simulink model "GS_model"  (R2018b)
settings: Solver=ode5  StartTime=0.0  StopTime=SimuStopTime  FixedStep=T_Simu  RelTol=1e-3
InitFcn:
  | Initial
undefined symbols (not defined in the file or in its folder): Aba10, Aba20, aeroCIP2006_S, aeroCIP2006_X, aeroCIP2006_Y, Agl0, Ass_kS, Ass_n1, Ass_n2, Ass_n3, Ass_n4, Ass_Noise, Ass_R, Ass_Resolution, Ass_TmOrder, AssA_Fix_Abs, AssB_Fix_Abs, AssC_Fix_Abs, AssD_Fix_Abs, AssE_Fix_Aps, AssF_Fix_Aps, C, c_max, c_min, Cd, CenterOfFigNX, CenterOfFigNY, CenterOfFigNZ, CenterOfFigP1, CenterOfFigP2, CenterOfFigPX, CenterOfFigPY, CenterOfFigPZ, Cmu, Crou, DEG2RAD, DiscIntNeverNeededParam, Eg_Dir, Eg_F, Eg_PrepareTime, Eg_r_L_L, Fw_Abf, Fw_Hmax, Fw_J, Fw_Spd0, Fw_Tmax, git_hash_BaseLine, git_hash_Project, Gnss_Noise_Pos, Gnss_Noise_Vel, Gnss_PropgationTime, GyroA_Fix_Abg, GyroA_Noise, GyroB_Fix_Abg, GyroB_Noise, GyroC_Fix_Abg, GyroC_Noise, GyroD_Fix_Abg, GyroD_Noise, h ... (+94)
libraries: simulink x308, sharedutil x46, aerolibutil x37, sharedtransform x31, vrlib x14, aerolibgravity2 x2
(part 17 of 20)

== system GS_model/Subsystem2/Subsystem/Sensor/Gyro/GyroBModel/GyroErrSet/GyroErrSet/GyroErrSet_Jump/Triggered Subsystem8 ==
  In1 : Inport
  Enable : EnablePort
  Out1 : Outport
  wires:
  In1/1 -> Out1/1

== system GS_model/Subsystem2/Subsystem/Sensor/Gyro/GyroBModel/GyroErrSet/GyroErrSet/GyroErrSet_Wave/Triggered Subsystem1 ==
  In1 : Inport
  Enable : EnablePort
  Out1 : Outport
  wires:
  In1/1 -> Out1/1

== system GS_model/Subsystem2/Subsystem/Sensor/Gyro/GyroBModel/GyroErrSet/GyroErrSet/GyroErrSet_Wave/Triggered Subsystem2 ==
  In1 : Inport
  Enable : EnablePort
  Out1 : Outport
  wires:
  In1/1 -> Out1/1

== system GS_model/Subsystem2/Subsystem/Sensor/Gyro/GyroBModel/GyroErrSet/GyroErrSet/GyroErrSet_Wave/Triggered Subsystem8 ==
  In1 : Inport
  Enable : EnablePort
  Out1 : Outport
  wires:
  In1/1 -> Out1/1

== system GS_model/Subsystem2/Subsystem/Sensor/Gyro/GyroBModel/GyroErrSet/GyroErrSet/GyroErrSet_WildValue/Triggered Subsystem1 ==
  In1 : Inport
  Enable : EnablePort
  Out1 : Outport
  wires:
  In1/1 -> Out1/1

== system GS_model/Subsystem2/Subsystem/Sensor/Gyro/GyroBModel/GyroErrSet/GyroErrSet/GyroErrSet_WildValue/Triggered Subsystem2 ==
  In1 : Inport
  Enable : EnablePort
  Out1 : Outport
  wires:
  In1/1 -> Out1/1

== system GS_model/Subsystem2/Subsystem/Sensor/Gyro/GyroBModel/GyroErrSet/GyroErrSet/GyroErrSet_WildValue/Triggered Subsystem8 ==
  In1 : Inport
  Enable : EnablePort
  Out1 : Outport
  wires:
  In1/1 -> Out1/1

== system GS_model/Subsystem2/Subsystem/Sensor/Gyro/GyroCModel/GyroErrSet/GyroErrSet/GyroErrSet_Constant/Triggered Subsystem1 ==
  In1 : Inport
  Enable : EnablePort
  Out1 : Outport
  wires:
  In1/1 -> Out1/1

== system GS_model/Subsystem2/Subsystem/Sensor/Gyro/GyroCModel/GyroErrSet/GyroErrSet/GyroErrSet_Constant/Triggered Subsystem2 ==
  In1 : Inport
  Enable : EnablePort
  Out1 : Outport
  wires:
  In1/1 -> Out1/1

== system GS_model/Subsystem2/Subsystem/Sensor/Gyro/GyroCModel/GyroErrSet/GyroErrSet/GyroErrSet_Constant/Triggered Subsystem8 ==
  In1 : Inport
  Enable : EnablePort
  Out1 : Outport
  wires:
  In1/1 -> Out1/1

== system GS_model/Subsystem2/Subsystem/Sensor/Gyro/GyroCModel/GyroErrSet/GyroErrSet/GyroErrSet_Jump/Triggered Subsystem1 ==
  In1 : Inport
  Enable : EnablePort
  Out1 : Outport
  wires:
  In1/1 -> Out1/1

== system GS_model/Subsystem2/Subsystem/Sensor/Gyro/GyroCModel/GyroErrSet/GyroErrSet/GyroErrSet_Jump/Triggered Subsystem2 ==
  In1 : Inport
  Enable : EnablePort
  Out1 : Outport
  wires:
  In1/1 -> Out1/1

== system GS_model/Subsystem2/Subsystem/Sensor/Gyro/GyroCModel/GyroErrSet/GyroErrSet/GyroErrSet_Jump/Triggered Subsystem8 ==
  In1 : Inport
  Enable : EnablePort
  Out1 : Outport
  wires:
  In1/1 -> Out1/1

== system GS_model/Subsystem2/Subsystem/Sensor/Gyro/GyroCModel/GyroErrSet/GyroErrSet/GyroErrSet_Wave/Triggered Subsystem1 ==
  In1 : Inport
  Enable : EnablePort
  Out1 : Outport
  wires:
  In1/1 -> Out1/1

== system GS_model/Subsystem2/Subsystem/Sensor/Gyro/GyroCModel/GyroErrSet/GyroErrSet/GyroErrSet_Wave/Triggered Subsystem2 ==
  In1 : Inport
  Enable : EnablePort
  Out1 : Outport
  wires:
  In1/1 -> Out1/1

== system GS_model/Subsystem2/Subsystem/Sensor/Gyro/GyroCModel/GyroErrSet/GyroErrSet/GyroErrSet_Wave/Triggered Subsystem8 ==
  In1 : Inport
  Enable : EnablePort
  Out1 : Outport
  wires:
  In1/1 -> Out1/1

== system GS_model/Subsystem2/Subsystem/Sensor/Gyro/GyroCModel/GyroErrSet/GyroErrSet/GyroErrSet_WildValue/Triggered Subsystem1 ==
  In1 : Inport
  Enable : EnablePort
  Out1 : Outport
  wires:
  In1/1 -> Out1/1

== system GS_model/Subsystem2/Subsystem/Sensor/Gyro/GyroCModel/GyroErrSet/GyroErrSet/GyroErrSet_WildValue/Triggered Subsystem2 ==
  In1 : Inport
  Enable : EnablePort
  Out1 : Outport
  wires:
  In1/1 -> Out1/1

== system GS_model/Subsystem2/Subsystem/Sensor/Gyro/GyroCModel/GyroErrSet/GyroErrSet/GyroErrSet_WildValue/Triggered Subsystem8 ==
  In1 : Inport
  Enable : EnablePort
  Out1 : Outport
  wires:
  In1/1 -> Out1/1

== system GS_model/Subsystem2/Subsystem/Sensor/Gyro/GyroDModel/GyroErrSet/GyroErrSet/GyroErrSet_Constant/Triggered Subsystem1 ==
  In1 : Inport
  Enable : EnablePort
  Out1 : Outport
  wires:
  In1/1 -> Out1/1

== system GS_model/Subsystem2/Subsystem/Sensor/Gyro/GyroDModel/GyroErrSet/GyroErrSet/GyroErrSet_Constant/Triggered Subsystem2 ==
  In1 : Inport
  Enable : EnablePort
  Out1 : Outport
  wires:
  In1/1 -> Out1/1

== system GS_model/Subsystem2/Subsystem/Sensor/Gyro/GyroDModel/GyroErrSet/GyroErrSet/GyroErrSet_Constant/Triggered Subsystem8 ==
  In1 : Inport
  Enable : EnablePort
  Out1 : Outport
  wires:
  In1/1 -> Out1/1

== system GS_model/Subsystem2/Subsystem/Sensor/Gyro/GyroDModel/GyroErrSet/GyroErrSet/GyroErrSet_Jump/Triggered Subsystem1 ==
  In1 : Inport
  Enable : EnablePort
  Out1 : Outport
  wires:
  In1/1 -> Out1/1

== system GS_model/Subsystem2/Subsystem/Sensor/Gyro/GyroDModel/GyroErrSet/GyroErrSet/GyroErrSet_Jump/Triggered Subsystem2 ==
  In1 : Inport
  Enable : EnablePort
  Out1 : Outport
  wires:
  In1/1 -> Out1/1

== system GS_model/Subsystem2/Subsystem/Sensor/Gyro/GyroDModel/GyroErrSet/GyroErrSet/GyroErrSet_Jump/Triggered Subsystem8 ==
  In1 : Inport
  Enable : EnablePort
  Out1 : Outport
  wires:
  In1/1 -> Out1/1

== system GS_model/Subsystem2/Subsystem/Sensor/Gyro/GyroDModel/GyroErrSet/GyroErrSet/GyroErrSet_Wave/Triggered Subsystem1 ==
  In1 : Inport
  Enable : EnablePort
  Out1 : Outport
  wires:
  In1/1 -> Out1/1

== system GS_model/Subsystem2/Subsystem/Sensor/Gyro/GyroDModel/GyroErrSet/GyroErrSet/GyroErrSet_Wave/Triggered Subsystem2 ==
  In1 : Inport
  Enable : EnablePort
  Out1 : Outport
  wires:
  In1/1 -> Out1/1

== system GS_model/Subsystem2/Subsystem/Sensor/Gyro/GyroDModel/GyroErrSet/GyroErrSet/GyroErrSet_Wave/Triggered Subsystem8 ==
  In1 : Inport
  Enable : EnablePort
  Out1 : Outport
  wires:
  In1/1 -> Out1/1

== system GS_model/Subsystem2/Subsystem/Sensor/Gyro/GyroDModel/GyroErrSet/GyroErrSet/GyroErrSet_WildValue/Triggered Subsystem1 ==
  In1 : Inport
  Enable : EnablePort
  Out1 : Outport
  wires:
  In1/1 -> Out1/1

== system GS_model/Subsystem2/Subsystem/Sensor/Gyro/GyroDModel/GyroErrSet/GyroErrSet/GyroErrSet_WildValue/Triggered Subsystem2 ==
  In1 : Inport
  Enable : EnablePort
  Out1 : Outport
  wires:
  In1/1 -> Out1/1

== system GS_model/Subsystem2/Subsystem/Sensor/Gyro/GyroDModel/GyroErrSet/GyroErrSet/GyroErrSet_WildValue/Triggered Subsystem8 ==
  In1 : Inport
  Enable : EnablePort
  Out1 : Outport
  wires:
  In1/1 -> Out1/1

== system GS_model/Subsystem2/Subsystem/Sensor/Magnetometer/MmModel1/Mm_ErrSet/MmErrSet/MmErrSet_Constant/MmAxisXErrSet_Constant ==
  MmAxis_in : Inport
  ErrSwitch : Inport  Port=2
  MmAxis_Num : Inport  Port=3
  Compare To Zero : simulink/Logic and Bit Operations/Compare To Zero  relop===  OutDataTypeStr=boolean
  Demux1 : Demux  Outputs=2
  Logical Operator : Logic  Operator=OR  AllPortsSameDT=off  OutDataTypeStr=boolean
  Memory : Memory
  Relational Operator9 : RelationalOperator  Operator===  OutDataTypeStr=boolean  RndMeth=Simplest
  Switch1 : Switch  Criteria=u2 > Threshold  Threshold=0.5
  Triggered Subsystem8 : Subsystem  TreatAsAtomicUnit=on
  MmAxis_out : Outport
  wires:
  Switch1/1 -> MmAxis_out/1, Memory/1
  MmAxis_in/1 -> Switch1/3
  Demux1/2 -> Triggered Subsystem8/1(In1)
  Memory/1 -> Switch1/1
  ErrSwitch/1 -> Demux1/1
  Triggered Subsystem8/1(Out1) -> Switch1/2
  Demux1/1 -> Compare To Zero/1, Relational Operator9/2
  MmAxis_Num/1 -> Relational Operator9/1
  Relational Operator9/1 -> Logical Operator/2
  Compare To Zero/1 -> Logical Operator/1
  Logical Operator/1 -> Triggered Subsystem8/Enable

== system GS_model/Subsystem2/Subsystem/Sensor/Magnetometer/MmModel1/Mm_ErrSet/MmErrSet/MmErrSet_Constant/MmAxisXErrSet_Constant1 ==
  MmAxis_in : Inport
  ErrSwitch : Inport  Port=2
  MmAxis_Num : Inport  Port=3
  Compare To Zero : simulink/Logic and Bit Operations/Compare To Zero  relop===  OutDataTypeStr=boolean
  Demux1 : Demux  Outputs=2
  Logical Operator : Logic  Operator=OR  AllPortsSameDT=off  OutDataTypeStr=boolean
  Memory : Memory
  Relational Operator9 : RelationalOperator  Operator===  OutDataTypeStr=boolean  RndMeth=Simplest
  Switch1 : Switch  Criteria=u2 > Threshold  Threshold=0.5
  Triggered Subsystem8 : Subsystem  TreatAsAtomicUnit=on
  MmAxis_out : Outport
  wires:
  Logical Operator/1 -> Triggered Subsystem8/Enable
  Compare To Zero/1 -> Logical Operator/1
  Relational Operator9/1 -> Logical Operator/2
  MmAxis_Num/1 -> Relational Operator9/1
  Demux1/1 -> Relational Operator9/2, Compare To Zero/1
  Triggered Subsystem8/1(Out1) -> Switch1/2
  ErrSwitch/1 -> Demux1/1
  Memory/1 -> Switch1/1
  Demux1/2 -> Triggered Subsystem8/1(In1)
  MmAxis_in/1 -> Switch1/3
  Switch1/1 -> Memory/1, MmAxis_out/1

== system GS_model/Subsystem2/Subsystem/Sensor/Magnetometer/MmModel1/Mm_ErrSet/MmErrSet/MmErrSet_Constant/MmAxisXErrSet_Constant2 ==
  MmAxis_in : Inport
  ErrSwitch : Inport  Port=2
  MmAxis_Num : Inport  Port=3
  Compare To Zero : simulink/Logic and Bit Operations/Compare To Zero  relop===  OutDataTypeStr=boolean
  Demux1 : Demux  Outputs=2
  Logical Operator : Logic  Operator=OR  AllPortsSameDT=off  OutDataTypeStr=boolean
  Memory : Memory
  Relational Operator9 : RelationalOperator  Operator===  OutDataTypeStr=boolean  RndMeth=Simplest
  Switch1 : Switch  Criteria=u2 > Threshold  Threshold=0.5
  Triggered Subsystem8 : Subsystem  TreatAsAtomicUnit=on
  MmAxis_out : Outport
  wires:
  Switch1/1 -> MmAxis_out/1, Memory/1
  MmAxis_in/1 -> Switch1/3
  Demux1/2 -> Triggered Subsystem8/1(In1)
  Memory/1 -> Switch1/1
  ErrSwitch/1 -> Demux1/1
  Triggered Subsystem8/1(Out1) -> Switch1/2
  Demux1/1 -> Compare To Zero/1, Relational Operator9/2
  MmAxis_Num/1 -> Relational Operator9/1
  Relational Operator9/1 -> Logical Operator/2
  Compare To Zero/1 -> Logical Operator/1
  Logical Operator/1 -> Triggered Subsystem8/Enable

== system GS_model/Subsystem2/Subsystem/Sensor/Magnetometer/MmModel1/Mm_ErrSet/MmErrSet/MmErrSet_Jump/MmAxisXErrSet_Jump ==
  MmAxis_in : Inport
  ErrSet : Inport  Port=2
  MmAxis_Num : Inport  Port=3
  MmAxis_JumpSet : Inport  Port=4
  Add : Sum  Inputs=|++
  Compare To Zero : simulink/Logic and Bit Operations/Compare To Zero  relop===  OutDataTypeStr=boolean
  Demux1 : Demux
  Logical Operator : Logic  Operator=OR  AllPortsSameDT=off  OutDataTypeStr=boolean
  Product : Product
  Relational Operator9 : RelationalOperator  Operator===  OutDataTypeStr=boolean  RndMeth=Simplest
  Switch3 : Switch  Criteria=u2 > Threshold  Threshold=0.5
  Terminator : Terminator
  Triggered Subsystem8 : Subsystem  TreatAsAtomicUnit=on
  MmAxis_out : Outport
  wires:
  MmAxis_JumpSet/1 -> Product/1
  Switch3/1 -> MmAxis_out/1
  MmAxis_Num/1 -> Relational Operator9/2
  Demux1/3 -> Terminator/1  "Period"
  Add/1 -> Switch3/1
  ErrSet/1 -> Demux1/1
  MmAxis_in/1 -> Add/2, Switch3/3
  Demux1/2 -> Triggered Subsystem8/1(In1)  "Switch"
  Product/1 -> Add/1
  Triggered Subsystem8/1(Out1) -> Switch3/2
  Demux1/4 -> Product/2  "Coff"
  Demux1/1 -> Compare To Zero/1, Relational Operator9/1  "Axis"
  Relational Operator9/1 -> Logical Operator/2
  Compare To Zero/1 -> Logical Operator/1
  Logical Operator/1 -> Triggered Subsystem8/Enable

== system GS_model/Subsystem2/Subsystem/Sensor/Magnetometer/MmModel1/Mm_ErrSet/MmErrSet/MmErrSet_Jump/MmAxisXErrSet_Jump1 ==
  MmAxis_in : Inport
  ErrSet : Inport  Port=2
  MmAxis_Num : Inport  Port=3
  MmAxis_JumpSet : Inport  Port=4
  Add : Sum  Inputs=|++
  Compare To Zero : simulink/Logic and Bit Operations/Compare To Zero  relop===  OutDataTypeStr=boolean
  Demux1 : Demux
  Logical Operator : Logic  Operator=OR  AllPortsSameDT=off  OutDataTypeStr=boolean
  Product : Product
  Relational Operator9 : RelationalOperator  Operator===  OutDataTypeStr=boolean  RndMeth=Simplest
  Switch3 : Switch  Criteria=u2 > Threshold  Threshold=0.5
  Terminator : Terminator
  Triggered Subsystem8 : Subsystem  TreatAsAtomicUnit=on
  MmAxis_out : Outport
  wires:
  Logical Operator/1 -> Triggered Subsystem8/Enable
  Compare To Zero/1 -> Logical Operator/1
  Relational Operator9/1 -> Logical Operator/2
  Demux1/1 -> Relational Operator9/1, Compare To Zero/1  "Axis"
  Demux1/4 -> Product/2  "Coff"
  Triggered Subsystem8/1(Out1) -> Switch3/2
  Product/1 -> Add/1
  Demux1/2 -> Triggered Subsystem8/1(In1)  "Switch"
  MmAxis_in/1 -> Switch3/3, Add/2
  ErrSet/1 -> Demux1/1
  Add/1 -> Switch3/1
  Demux1/3 -> Terminator/1  "Period"
  MmAxis_Num/1 -> Relational Operator9/2
  Switch3/1 -> MmAxis_out/1
  MmAxis_JumpSet/1 -> Product/1

== system GS_model/Subsystem2/Subsystem/Sensor/Magnetometer/MmModel1/Mm_ErrSet/MmErrSet/MmErrSet_Jump/MmAxisXErrSet_Jump2 ==
  MmAxis_in : Inport
  ErrSet : Inport  Port=2
  MmAxis_Num : Inport  Port=3
  MmAxis_JumpSet : Inport  Port=4
  Add : Sum  Inputs=|++
  Compare To Zero : simulink/Logic and Bit Operations/Compare To Zero  relop===  OutDataTypeStr=boolean
  Demux1 : Demux
  Logical Operator : Logic  Operator=OR  AllPortsSameDT=off  OutDataTypeStr=boolean
  Product : Product
  Relational Operator9 : RelationalOperator  Operator===  OutDataTypeStr=boolean  RndMeth=Simplest
  Switch3 : Switch  Criteria=u2 > Threshold  Threshold=0.5
  Terminator : Terminator
  Triggered Subsystem8 : Subsystem  TreatAsAtomicUnit=on
  MmAxis_out : Outport
  wires:
  MmAxis_JumpSet/1 -> Product/1
  Switch3/1 -> MmAxis_out/1
  MmAxis_Num/1 -> Relational Operator9/2
  Demux1/3 -> Terminator/1  "Period"
  Add/1 -> Switch3/1
  ErrSet/1 -> Demux1/1
  MmAxis_in/1 -> Add/2, Switch3/3
  Demux1/2 -> Triggered Subsystem8/1(In1)  "Switch"
  Product/1 -> Add/1
  Triggered Subsystem8/1(Out1) -> Switch3/2
  Demux1/4 -> Product/2  "Coff"
  Demux1/1 -> Compare To Zero/1, Relational Operator9/1  "Axis"
  Relational Operator9/1 -> Logical Operator/2
  Compare To Zero/1 -> Logical Operator/1
  Logical Operator/1 -> Triggered Subsystem8/Enable

== system GS_model/Subsystem2/Subsystem/Sensor/Magnetometer/MmModel1/Mm_ErrSet/MmErrSet/MmErrSet_Wave/MmAxisXErrSet_Wave ==
  MmAxis_in : Inport
  ErrSet : Inport  Port=2
  MmAxis_Num : Inport  Port=3
  MmAxis_WaveSet : Inport  Port=4
  Add : Sum  Inputs=|++
  Compare To Zero : simulink/Logic and Bit Operations/Compare To Zero  relop===  OutDataTypeStr=boolean
  Demux1 : Demux  Outputs=3
  Logical Operator : Logic  Operator=OR  AllPortsSameDT=off  OutDataTypeStr=boolean
  Product : Product
  Relational Operator9 : RelationalOperator  Operator===  OutDataTypeStr=boolean  RndMeth=Simplest
  Switch3 : Switch  Criteria=u2 > Threshold  Threshold=0.5
  Triggered Subsystem8 : Subsystem  TreatAsAtomicUnit=on
  MmAxis_out : Outport
  wires:
  Triggered Subsystem8/1(Out1) -> Switch3/2
  Switch3/1 -> MmAxis_out/1
  MmAxis_Num/1 -> Relational Operator9/2
  Demux1/3 -> Product/2  "Coff"
  Demux1/1 -> Compare To Zero/1, Relational Operator9/1  "Axis"
  Demux1/2 -> Triggered Subsystem8/1(In1)  "Switch"
  MmAxis_in/1 -> Switch3/3, Add/2
  Add/1 -> Switch3/1
  ErrSet/1 -> Demux1/1
  Product/1 -> Add/1
  MmAxis_WaveSet/1 -> Product/1
  Relational Operator9/1 -> Logical Operator/2
  Logical Operator/1 -> Triggered Subsystem8/Enable
  Compare To Zero/1 -> Logical Operator/1

== system GS_model/Subsystem2/Subsystem/Sensor/Magnetometer/MmModel1/Mm_ErrSet/MmErrSet/MmErrSet_Wave/MmAxisXErrSet_Wave1 ==
  MmAxis_in : Inport
  ErrSet : Inport  Port=2
  MmAxis_Num : Inport  Port=3
  MmAxis_WaveSet : Inport  Port=4
  Add : Sum  Inputs=|++
  Compare To Zero : simulink/Logic and Bit Operations/Compare To Zero  relop===  OutDataTypeStr=boolean
  Demux1 : Demux  Outputs=3
  Logical Operator : Logic  Operator=OR  AllPortsSameDT=off  OutDataTypeStr=boolean
  Product : Product
  Relational Operator9 : RelationalOperator  Operator===  OutDataTypeStr=boolean  RndMeth=Simplest
  Switch3 : Switch  Criteria=u2 > Threshold  Threshold=0.5
  Triggered Subsystem8 : Subsystem  TreatAsAtomicUnit=on
  MmAxis_out : Outport
  wires:
  Compare To Zero/1 -> Logical Operator/1
  Logical Operator/1 -> Triggered Subsystem8/Enable
  Relational Operator9/1 -> Logical Operator/2
  MmAxis_WaveSet/1 -> Product/1
  Product/1 -> Add/1
  ErrSet/1 -> Demux1/1
  Add/1 -> Switch3/1
  MmAxis_in/1 -> Add/2, Switch3/3
  Demux1/2 -> Triggered Subsystem8/1(In1)  "Switch"
  Demux1/1 -> Relational Operator9/1, Compare To Zero/1  "Axis"
  Demux1/3 -> Product/2  "Coff"
  MmAxis_Num/1 -> Relational Operator9/2
  Switch3/1 -> MmAxis_out/1
  Triggered Subsystem8/1(Out1) -> Switch3/2

== system GS_model/Subsystem2/Subsystem/Sensor/Magnetometer/MmModel1/Mm_ErrSet/MmErrSet/MmErrSet_Wave/MmAxisXErrSet_Wave2 ==
  MmAxis_in : Inport
  ErrSet : Inport  Port=2
  MmAxis_Num : Inport  Port=3
  MmAxis_WaveSet : Inport  Port=4
  Add : Sum  Inputs=|++
  Compare To Zero : simulink/Logic and Bit Operations/Compare To Zero  relop===  OutDataTypeStr=boolean
  Demux1 : Demux  Outputs=3
  Logical Operator : Logic  Operator=OR  AllPortsSameDT=off  OutDataTypeStr=boolean
  Product : Product
  Relational Operator9 : RelationalOperator  Operator===  OutDataTypeStr=boolean  RndMeth=Simplest
  Switch3 : Switch  Criteria=u2 > Threshold  Threshold=0.5
  Triggered Subsystem8 : Subsystem  TreatAsAtomicUnit=on
  MmAxis_out : Outport
  wires:
  Triggered Subsystem8/1(Out1) -> Switch3/2
  Switch3/1 -> MmAxis_out/1
  MmAxis_Num/1 -> Relational Operator9/2
  Demux1/3 -> Product/2  "Coff"
  Demux1/1 -> Compare To Zero/1, Relational Operator9/1  "Axis"
  Demux1/2 -> Triggered Subsystem8/1(In1)  "Switch"
  MmAxis_in/1 -> Switch3/3, Add/2
  Add/1 -> Switch3/1
  ErrSet/1 -> Demux1/1
  Product/1 -> Add/1
  MmAxis_WaveSet/1 -> Product/1
  Relational Operator9/1 -> Logical Operator/2
  Logical Operator/1 -> Triggered Subsystem8/Enable
  Compare To Zero/1 -> Logical Operator/1

== system GS_model/Subsystem2/Subsystem/Sensor/Magnetometer/MmModel1/Mm_ErrSet/MmErrSet/MmErrSet_WildValue/MmAxisXErrSet_WildValue ==
  MmAxis_in : Inport
  ErrSwitch : Inport  Port=2
  MmAxis_Num : Inport  Port=3
  MmAxis_WildValue : Inport  Port=4
  Compare To Zero : simulink/Logic and Bit Operations/Compare To Zero  relop===  OutDataTypeStr=boolean
  Demux1 : Demux  Outputs=2
  Logical Operator : Logic  Operator=OR  AllPortsSameDT=off  OutDataTypeStr=boolean
  Relational Operator9 : RelationalOperator  Operator===  OutDataTypeStr=boolean  RndMeth=Simplest
  Switch1 : Switch  Criteria=u2 > Threshold  Threshold=0.5
  Triggered Subsystem8 : Subsystem  TreatAsAtomicUnit=on
  MmAxis_out : Outport
  wires:
  ErrSwitch/1 -> Demux1/1
  MmAxis_WildValue/1 -> Switch1/1
  MmAxis_Num/1 -> Relational Operator9/2
  Triggered Subsystem8/1(Out1) -> Switch1/2
  Demux1/2 -> Triggered Subsystem8/1(In1)
  Demux1/1 -> Compare To Zero/1, Relational Operator9/1
  MmAxis_in/1 -> Switch1/3
  Switch1/1 -> MmAxis_out/1
  Relational Operator9/1 -> Logical Operator/2
  Compare To Zero/1 -> Logical Operator/1
  Logical Operator/1 -> Triggered Subsystem8/Enable

== system GS_model/Subsystem2/Subsystem/Sensor/Magnetometer/MmModel1/Mm_ErrSet/MmErrSet/MmErrSet_WildValue/MmAxisXErrSet_WildValue1 ==
  MmAxis_in : Inport
  ErrSwitch : Inport  Port=2
  MmAxis_Num : Inport  Port=3
  MmAxis_WildValue : Inport  Port=4
  Compare To Zero : simulink/Logic and Bit Operations/Compare To Zero  relop===  OutDataTypeStr=boolean
  Demux1 : Demux  Outputs=2
  Logical Operator : Logic  Operator=OR  AllPortsSameDT=off  OutDataTypeStr=boolean
  Relational Operator9 : RelationalOperator  Operator===  OutDataTypeStr=boolean  RndMeth=Simplest
  Switch1 : Switch  Criteria=u2 > Threshold  Threshold=0.5
  Triggered Subsystem8 : Subsystem  TreatAsAtomicUnit=on
  MmAxis_out : Outport
  wires:
  Logical Operator/1 -> Triggered Subsystem8/Enable
  Compare To Zero/1 -> Logical Operator/1
  Relational Operator9/1 -> Logical Operator/2
  Switch1/1 -> MmAxis_out/1
  MmAxis_in/1 -> Switch1/3
  Demux1/1 -> Relational Operator9/1, Compare To Zero/1
  Demux1/2 -> Triggered Subsystem8/1(In1)
  Triggered Subsystem8/1(Out1) -> Switch1/2
  MmAxis_Num/1 -> Relational Operator9/2
  MmAxis_WildValue/1 -> Switch1/1
  ErrSwitch/1 -> Demux1/1

== system GS_model/Subsystem2/Subsystem/Sensor/Magnetometer/MmModel1/Mm_ErrSet/MmErrSet/MmErrSet_WildValue/MmAxisXErrSet_WildValue2 ==
  MmAxis_in : Inport
  ErrSwitch : Inport  Port=2
  MmAxis_Num : Inport  Port=3
  MmAxis_WildValue : Inport  Port=4
  Compare To Zero : simulink/Logic and Bit Operations/Compare To Zero  relop===  OutDataTypeStr=boolean
  Demux1 : Demux  Outputs=2
  Logical Operator : Logic  Operator=OR  AllPortsSameDT=off  OutDataTypeStr=boolean
  Relational Operator9 : RelationalOperator  Operator===  OutDataTypeStr=boolean  RndMeth=Simplest
  Switch1 : Switch  Criteria=u2 > Threshold  Threshold=0.5
  Triggered Subsystem8 : Subsystem  TreatAsAtomicUnit=on
  MmAxis_out : Outport
  wires:
  ErrSwitch/1 -> Demux1/1
  MmAxis_WildValue/1 -> Switch1/1
  MmAxis_Num/1 -> Relational Operator9/2
  Triggered Subsystem8/1(Out1) -> Switch1/2
  Demux1/2 -> Triggered Subsystem8/1(In1)
  Demux1/1 -> Compare To Zero/1, Relational Operator9/1
  MmAxis_in/1 -> Switch1/3
  Switch1/1 -> MmAxis_out/1
  Relational Operator9/1 -> Logical Operator/2
  Compare To Zero/1 -> Logical Operator/1
  Logical Operator/1 -> Triggered Subsystem8/Enable

== system GS_model/Subsystem2/Subsystem/Sensor/Magnetometer/MmModel2/Mm_ErrSet/MmErrSet/MmErrSet_Constant/MmAxisXErrSet_Constant ==
  MmAxis_in : Inport
  ErrSwitch : Inport  Port=2
  MmAxis_Num : Inport  Port=3
  Compare To Zero : simulink/Logic and Bit Operations/Compare To Zero  relop===  OutDataTypeStr=boolean
  Demux1 : Demux  Outputs=2
  Logical Operator : Logic  Operator=OR  AllPortsSameDT=off  OutDataTypeStr=boolean
  Memory : Memory
  Relational Operator9 : RelationalOperator  Operator===  OutDataTypeStr=boolean  RndMeth=Simplest
  Switch1 : Switch  Criteria=u2 > Threshold  Threshold=0.5
  Triggered Subsystem8 : Subsystem  TreatAsAtomicUnit=on
  MmAxis_out : Outport
  wires:
  Logical Operator/1 -> Triggered Subsystem8/Enable
  Compare To Zero/1 -> Logical Operator/1
  Relational Operator9/1 -> Logical Operator/2
  MmAxis_Num/1 -> Relational Operator9/1
  Demux1/1 -> Relational Operator9/2, Compare To Zero/1
  Triggered Subsystem8/1(Out1) -> Switch1/2
  ErrSwitch/1 -> Demux1/1
  Memory/1 -> Switch1/1
  Demux1/2 -> Triggered Subsystem8/1(In1)
  MmAxis_in/1 -> Switch1/3
  Switch1/1 -> Memory/1, MmAxis_out/1

== system GS_model/Subsystem2/Subsystem/Sensor/Magnetometer/MmModel2/Mm_ErrSet/MmErrSet/MmErrSet_Constant/MmAxisXErrSet_Constant1 ==
  MmAxis_in : Inport
  ErrSwitch : Inport  Port=2
  MmAxis_Num : Inport  Port=3
  Compare To Zero : simulink/Logic and Bit Operations/Compare To Zero  relop===  OutDataTypeStr=boolean
  Demux1 : Demux  Outputs=2
  Logical Operator : Logic  Operator=OR  AllPortsSameDT=off  OutDataTypeStr=boolean
  Memory : Memory
  Relational Operator9 : RelationalOperator  Operator===  OutDataTypeStr=boolean  RndMeth=Simplest
  Switch1 : Switch  Criteria=u2 > Threshold  Threshold=0.5
  Triggered Subsystem8 : Subsystem  TreatAsAtomicUnit=on
  MmAxis_out : Outport
  wires:
  Switch1/1 -> MmAxis_out/1, Memory/1
  MmAxis_in/1 -> Switch1/3
  Demux1/2 -> Triggered Subsystem8/1(In1)
  Memory/1 -> Switch1/1
  ErrSwitch/1 -> Demux1/1
  Triggered Subsystem8/1(Out1) -> Switch1/2
  Demux1/1 -> Compare To Zero/1, Relational Operator9/2
  MmAxis_Num/1 -> Relational Operator9/1
  Relational Operator9/1 -> Logical Operator/2
  Compare To Zero/1 -> Logical Operator/1
  Logical Operator/1 -> Triggered Subsystem8/Enable

== system GS_model/Subsystem2/Subsystem/Sensor/Magnetometer/MmModel2/Mm_ErrSet/MmErrSet/MmErrSet_Constant/MmAxisXErrSet_Constant2 ==
  MmAxis_in : Inport
  ErrSwitch : Inport  Port=2
  MmAxis_Num : Inport  Port=3
  Compare To Zero : simulink/Logic and Bit Operations/Compare To Zero  relop===  OutDataTypeStr=boolean
  Demux1 : Demux  Outputs=2
  Logical Operator : Logic  Operator=OR  AllPortsSameDT=off  OutDataTypeStr=boolean
  Memory : Memory
  Relational Operator9 : RelationalOperator  Operator===  OutDataTypeStr=boolean  RndMeth=Simplest
  Switch1 : Switch  Criteria=u2 > Threshold  Threshold=0.5
  Triggered Subsystem8 : Subsystem  TreatAsAtomicUnit=on
  MmAxis_out : Outport
  wires:
  Logical Operator/1 -> Triggered Subsystem8/Enable
  Compare To Zero/1 -> Logical Operator/1
  Relational Operator9/1 -> Logical Operator/2
  MmAxis_Num/1 -> Relational Operator9/1
  Demux1/1 -> Relational Operator9/2, Compare To Zero/1
  Triggered Subsystem8/1(Out1) -> Switch1/2
  ErrSwitch/1 -> Demux1/1
  Memory/1 -> Switch1/1
  Demux1/2 -> Triggered Subsystem8/1(In1)
  MmAxis_in/1 -> Switch1/3
  Switch1/1 -> Memory/1, MmAxis_out/1

== system GS_model/Subsystem2/Subsystem/Sensor/Magnetometer/MmModel2/Mm_ErrSet/MmErrSet/MmErrSet_Jump/MmAxisXErrSet_Jump ==
  MmAxis_in : Inport
  ErrSet : Inport  Port=2
  MmAxis_Num : Inport  Port=3
  MmAxis_JumpSet : Inport  Port=4
  Add : Sum  Inputs=|++
  Compare To Zero : simulink/Logic and Bit Operations/Compare To Zero  relop===  OutDataTypeStr=boolean
  Demux1 : Demux
  Logical Operator : Logic  Operator=OR  AllPortsSameDT=off  OutDataTypeStr=boolean
  Product : Product
  Relational Operator9 : RelationalOperator  Operator===  OutDataTypeStr=boolean  RndMeth=Simplest
  Switch3 : Switch  Criteria=u2 > Threshold  Threshold=0.5
  Terminator : Terminator
  Triggered Subsystem8 : Subsystem  TreatAsAtomicUnit=on
  MmAxis_out : Outport
  wires:
  Logical Operator/1 -> Triggered Subsystem8/Enable
  Compare To Zero/1 -> Logical Operator/1
  Relational Operator9/1 -> Logical Operator/2
  Demux1/1 -> Relational Operator9/1, Compare To Zero/1  "Axis"
  Demux1/4 -> Product/2  "Coff"
  Triggered Subsystem8/1(Out1) -> Switch3/2
  Product/1 -> Add/1
  Demux1/2 -> Triggered Subsystem8/1(In1)  "Switch"
  MmAxis_in/1 -> Switch3/3, Add/2
  ErrSet/1 -> Demux1/1
  Add/1 -> Switch3/1
  Demux1/3 -> Terminator/1  "Period"
  MmAxis_Num/1 -> Relational Operator9/2
  Switch3/1 -> MmAxis_out/1
  MmAxis_JumpSet/1 -> Product/1

== system GS_model/Subsystem2/Subsystem/Sensor/Magnetometer/MmModel2/Mm_ErrSet/MmErrSet/MmErrSet_Jump/MmAxisXErrSet_Jump1 ==
  MmAxis_in : Inport
  ErrSet : Inport  Port=2
  MmAxis_Num : Inport  Port=3
  MmAxis_JumpSet : Inport  Port=4
  Add : Sum  Inputs=|++
  Compare To Zero : simulink/Logic and Bit Operations/Compare To Zero  relop===  OutDataTypeStr=boolean
  Demux1 : Demux
  Logical Operator : Logic  Operator=OR  AllPortsSameDT=off  OutDataTypeStr=boolean
  Product : Product
  Relational Operator9 : RelationalOperator  Operator===  OutDataTypeStr=boolean  RndMeth=Simplest
  Switch3 : Switch  Criteria=u2 > Threshold  Threshold=0.5
  Terminator : Terminator
  Triggered Subsystem8 : Subsystem  TreatAsAtomicUnit=on
  MmAxis_out : Outport
  wires:
  MmAxis_JumpSet/1 -> Product/1
  Switch3/1 -> MmAxis_out/1
  MmAxis_Num/1 -> Relational Operator9/2
  Demux1/3 -> Terminator/1  "Period"
  Add/1 -> Switch3/1
  ErrSet/1 -> Demux1/1
  MmAxis_in/1 -> Add/2, Switch3/3
  Demux1/2 -> Triggered Subsystem8/1(In1)  "Switch"
  Product/1 -> Add/1
  Triggered Subsystem8/1(Out1) -> Switch3/2
  Demux1/4 -> Product/2  "Coff"
  Demux1/1 -> Compare To Zero/1, Relational Operator9/1  "Axis"
  Relational Operator9/1 -> Logical Operator/2
  Compare To Zero/1 -> Logical Operator/1
  Logical Operator/1 -> Triggered Subsystem8/Enable

== system GS_model/Subsystem2/Subsystem/Sensor/Magnetometer/MmModel2/Mm_ErrSet/MmErrSet/MmErrSet_Jump/MmAxisXErrSet_Jump2 ==
  MmAxis_in : Inport
  ErrSet : Inport  Port=2
  MmAxis_Num : Inport  Port=3
  MmAxis_JumpSet : Inport  Port=4
  Add : Sum  Inputs=|++
  Compare To Zero : simulink/Logic and Bit Operations/Compare To Zero  relop===  OutDataTypeStr=boolean
  Demux1 : Demux
  Logical Operator : Logic  Operator=OR  AllPortsSameDT=off  OutDataTypeStr=boolean
  Product : Product
  Relational Operator9 : RelationalOperator  Operator===  OutDataTypeStr=boolean  RndMeth=Simplest
  Switch3 : Switch  Criteria=u2 > Threshold  Threshold=0.5
  Terminator : Terminator
  Triggered Subsystem8 : Subsystem  TreatAsAtomicUnit=on
  MmAxis_out : Outport
  wires:
  Logical Operator/1 -> Triggered Subsystem8/Enable
  Compare To Zero/1 -> Logical Operator/1
  Relational Operator9/1 -> Logical Operator/2
  Demux1/1 -> Relational Operator9/1, Compare To Zero/1  "Axis"
  Demux1/4 -> Product/2  "Coff"
  Triggered Subsystem8/1(Out1) -> Switch3/2
  Product/1 -> Add/1
  Demux1/2 -> Triggered Subsystem8/1(In1)  "Switch"
  MmAxis_in/1 -> Switch3/3, Add/2
  ErrSet/1 -> Demux1/1
  Add/1 -> Switch3/1
  Demux1/3 -> Terminator/1  "Period"
  MmAxis_Num/1 -> Relational Operator9/2
  Switch3/1 -> MmAxis_out/1
  MmAxis_JumpSet/1 -> Product/1

== system GS_model/Subsystem2/Subsystem/Sensor/Magnetometer/MmModel2/Mm_ErrSet/MmErrSet/MmErrSet_Wave/MmAxisXErrSet_Wave ==
  MmAxis_in : Inport
  ErrSet : Inport  Port=2
  MmAxis_Num : Inport  Port=3
  MmAxis_WaveSet : Inport  Port=4
  Add : Sum  Inputs=|++
  Compare To Zero : simulink/Logic and Bit Operations/Compare To Zero  relop===  OutDataTypeStr=boolean
  Demux1 : Demux  Outputs=3
  Logical Operator : Logic  Operator=OR  AllPortsSameDT=off  OutDataTypeStr=boolean
  Product : Product
  Relational Operator9 : RelationalOperator  Operator===  OutDataTypeStr=boolean  RndMeth=Simplest
  Switch3 : Switch  Criteria=u2 > Threshold  Threshold=0.5
  Triggered Subsystem8 : Subsystem  TreatAsAtomicUnit=on
  MmAxis_out : Outport
  wires:
  Compare To Zero/1 -> Logical Operator/1
  Logical Operator/1 -> Triggered Subsystem8/Enable
  Relational Operator9/1 -> Logical Operator/2
  MmAxis_WaveSet/1 -> Product/1
  Product/1 -> Add/1
  ErrSet/1 -> Demux1/1
  Add/1 -> Switch3/1
  MmAxis_in/1 -> Add/2, Switch3/3
  Demux1/2 -> Triggered Subsystem8/1(In1)  "Switch"
  Demux1/1 -> Relational Operator9/1, Compare To Zero/1  "Axis"
  Demux1/3 -> Product/2  "Coff"
  MmAxis_Num/1 -> Relational Operator9/2
  Switch3/1 -> MmAxis_out/1
  Triggered Subsystem8/1(Out1) -> Switch3/2

== system GS_model/Subsystem2/Subsystem/Sensor/Magnetometer/MmModel2/Mm_ErrSet/MmErrSet/MmErrSet_Wave/MmAxisXErrSet_Wave1 ==
  MmAxis_in : Inport
  ErrSet : Inport  Port=2
  MmAxis_Num : Inport  Port=3
  MmAxis_WaveSet : Inport  Port=4
  Add : Sum  Inputs=|++
  Compare To Zero : simulink/Logic and Bit Operations/Compare To Zero  relop===  OutDataTypeStr=boolean
  Demux1 : Demux  Outputs=3
  Logical Operator : Logic  Operator=OR  AllPortsSameDT=off  OutDataTypeStr=boolean
  Product : Product
  Relational Operator9 : RelationalOperator  Operator===  OutDataTypeStr=boolean  RndMeth=Simplest
  Switch3 : Switch  Criteria=u2 > Threshold  Threshold=0.5
  Triggered Subsystem8 : Subsystem  TreatAsAtomicUnit=on
  MmAxis_out : Outport
  wires:
  Triggered Subsystem8/1(Out1) -> Switch3/2
  Switch3/1 -> MmAxis_out/1
  MmAxis_Num/1 -> Relational Operator9/2
  Demux1/3 -> Product/2  "Coff"
  Demux1/1 -> Compare To Zero/1, Relational Operator9/1  "Axis"
  Demux1/2 -> Triggered Subsystem8/1(In1)  "Switch"
  MmAxis_in/1 -> Switch3/3, Add/2
  Add/1 -> Switch3/1
  ErrSet/1 -> Demux1/1
  Product/1 -> Add/1
  MmAxis_WaveSet/1 -> Product/1
  Relational Operator9/1 -> Logical Operator/2
  Logical Operator/1 -> Triggered Subsystem8/Enable
  Compare To Zero/1 -> Logical Operator/1

== system GS_model/Subsystem2/Subsystem/Sensor/Magnetometer/MmModel2/Mm_ErrSet/MmErrSet/MmErrSet_Wave/MmAxisXErrSet_Wave2 ==
  MmAxis_in : Inport
  ErrSet : Inport  Port=2
  MmAxis_Num : Inport  Port=3
  MmAxis_WaveSet : Inport  Port=4
  Add : Sum  Inputs=|++
  Compare To Zero : simulink/Logic and Bit Operations/Compare To Zero  relop===  OutDataTypeStr=boolean
  Demux1 : Demux  Outputs=3
  Logical Operator : Logic  Operator=OR  AllPortsSameDT=off  OutDataTypeStr=boolean
  Product : Product
  Relational Operator9 : RelationalOperator  Operator===  OutDataTypeStr=boolean  RndMeth=Simplest
  Switch3 : Switch  Criteria=u2 > Threshold  Threshold=0.5
  Triggered Subsystem8 : Subsystem  TreatAsAtomicUnit=on
  MmAxis_out : Outport
  wires:
  Compare To Zero/1 -> Logical Operator/1
  Logical Operator/1 -> Triggered Subsystem8/Enable
  Relational Operator9/1 -> Logical Operator/2
  MmAxis_WaveSet/1 -> Product/1
  Product/1 -> Add/1
  ErrSet/1 -> Demux1/1
  Add/1 -> Switch3/1
  MmAxis_in/1 -> Add/2, Switch3/3
  Demux1/2 -> Triggered Subsystem8/1(In1)  "Switch"
  Demux1/1 -> Relational Operator9/1, Compare To Zero/1  "Axis"
  Demux1/3 -> Product/2  "Coff"
  MmAxis_Num/1 -> Relational Operator9/2
  Switch3/1 -> MmAxis_out/1
  Triggered Subsystem8/1(Out1) -> Switch3/2

== system GS_model/Subsystem2/Subsystem/Sensor/Magnetometer/MmModel2/Mm_ErrSet/MmErrSet/MmErrSet_WildValue/MmAxisXErrSet_WildValue ==
  MmAxis_in : Inport
  ErrSwitch : Inport  Port=2
  MmAxis_Num : Inport  Port=3
  MmAxis_WildValue : Inport  Port=4
  Compare To Zero : simulink/Logic and Bit Operations/Compare To Zero  relop===  OutDataTypeStr=boolean
  Demux1 : Demux  Outputs=2
  Logical Operator : Logic  Operator=OR  AllPortsSameDT=off  OutDataTypeStr=boolean
  Relational Operator9 : RelationalOperator  Operator===  OutDataTypeStr=boolean  RndMeth=Simplest
  Switch1 : Switch  Criteria=u2 > Threshold  Threshold=0.5
  Triggered Subsystem8 : Subsystem  TreatAsAtomicUnit=on
  MmAxis_out : Outport
  wires:
  Logical Operator/1 -> Triggered Subsystem8/Enable
  Compare To Zero/1 -> Logical Operator/1
  Relational Operator9/1 -> Logical Operator/2
  Switch1/1 -> MmAxis_out/1
  MmAxis_in/1 -> Switch1/3
  Demux1/1 -> Relational Operator9/1, Compare To Zero/1
  Demux1/2 -> Triggered Subsystem8/1(In1)
  Triggered Subsystem8/1(Out1) -> Switch1/2
  MmAxis_Num/1 -> Relational Operator9/2
  MmAxis_WildValue/1 -> Switch1/1
  ErrSwitch/1 -> Demux1/1

== system GS_model/Subsystem2/Subsystem/Sensor/Magnetometer/MmModel2/Mm_ErrSet/MmErrSet/MmErrSet_WildValue/MmAxisXErrSet_WildValue1 ==
  MmAxis_in : Inport
  ErrSwitch : Inport  Port=2
  MmAxis_Num : Inport  Port=3
  MmAxis_WildValue : Inport  Port=4
  Compare To Zero : simulink/Logic and Bit Operations/Compare To Zero  relop===  OutDataTypeStr=boolean
  Demux1 : Demux  Outputs=2
  Logical Operator : Logic  Operator=OR  AllPortsSameDT=off  OutDataTypeStr=boolean
  Relational Operator9 : RelationalOperator  Operator===  OutDataTypeStr=boolean  RndMeth=Simplest
  Switch1 : Switch  Criteria=u2 > Threshold  Threshold=0.5
  Triggered Subsystem8 : Subsystem  TreatAsAtomicUnit=on
  MmAxis_out : Outport
  wires:
  ErrSwitch/1 -> Demux1/1
  MmAxis_WildValue/1 -> Switch1/1
  MmAxis_Num/1 -> Relational Operator9/2
  Triggered Subsystem8/1(Out1) -> Switch1/2
  Demux1/2 -> Triggered Subsystem8/1(In1)
  Demux1/1 -> Compare To Zero/1, Relational Operator9/1
  MmAxis_in/1 -> Switch1/3
  Switch1/1 -> MmAxis_out/1
  Relational Operator9/1 -> Logical Operator/2
  Compare To Zero/1 -> Logical Operator/1
  Logical Operator/1 -> Triggered Subsystem8/Enable

== system GS_model/Subsystem2/Subsystem/Sensor/Magnetometer/MmModel2/Mm_ErrSet/MmErrSet/MmErrSet_WildValue/MmAxisXErrSet_WildValue2 ==
  MmAxis_in : Inport
  ErrSwitch : Inport  Port=2
  MmAxis_Num : Inport  Port=3
  MmAxis_WildValue : Inport  Port=4
  Compare To Zero : simulink/Logic and Bit Operations/Compare To Zero  relop===  OutDataTypeStr=boolean
  Demux1 : Demux  Outputs=2
  Logical Operator : Logic  Operator=OR  AllPortsSameDT=off  OutDataTypeStr=boolean
  Relational Operator9 : RelationalOperator  Operator===  OutDataTypeStr=boolean  RndMeth=Simplest
  Switch1 : Switch  Criteria=u2 > Threshold  Threshold=0.5
  Triggered Subsystem8 : Subsystem  TreatAsAtomicUnit=on
  MmAxis_out : Outport
  wires:
  Logical Operator/1 -> Triggered Subsystem8/Enable
  Compare To Zero/1 -> Logical Operator/1
  Relational Operator9/1 -> Logical Operator/2
  Switch1/1 -> MmAxis_out/1
  MmAxis_in/1 -> Switch1/3
  Demux1/1 -> Relational Operator9/1, Compare To Zero/1
  Demux1/2 -> Triggered Subsystem8/1(In1)
  Triggered Subsystem8/1(Out1) -> Switch1/2
  MmAxis_Num/1 -> Relational Operator9/2
  MmAxis_WildValue/1 -> Switch1/1
  ErrSwitch/1 -> Demux1/1

== system GS_model/Subsystem2/Subsystem/Sensor/Magnetometer/MmModel3/Mm_ErrSet/MmErrSet/MmErrSet_Constant/MmAxisXErrSet_Constant ==
  MmAxis_in : Inport
  ErrSwitch : Inport  Port=2
  MmAxis_Num : Inport  Port=3
  Compare To Zero : simulink/Logic and Bit Operations/Compare To Zero  relop===  OutDataTypeStr=boolean
  Demux1 : Demux  Outputs=2
  Logical Operator : Logic  Operator=OR  AllPortsSameDT=off  OutDataTypeStr=boolean
  Memory : Memory
  Relational Operator9 : RelationalOperator  Operator===  OutDataTypeStr=boolean  RndMeth=Simplest
  Switch1 : Switch  Criteria=u2 > Threshold  Threshold=0.5
  Triggered Subsystem8 : Subsystem  TreatAsAtomicUnit=on
  MmAxis_out : Outport
  wires:
  Switch1/1 -> MmAxis_out/1, Memory/1
  MmAxis_in/1 -> Switch1/3
  Demux1/2 -> Triggered Subsystem8/1(In1)
  Memory/1 -> Switch1/1
  ErrSwitch/1 -> Demux1/1
  Triggered Subsystem8/1(Out1) -> Switch1/2
  Demux1/1 -> Compare To Zero/1, Relational Operator9/2
  MmAxis_Num/1 -> Relational Operator9/1
  Relational Operator9/1 -> Logical Operator/2
  Compare To Zero/1 -> Logical Operator/1
  Logical Operator/1 -> Triggered Subsystem8/Enable

== system GS_model/Subsystem2/Subsystem/Sensor/Magnetometer/MmModel3/Mm_ErrSet/MmErrSet/MmErrSet_Constant/MmAxisXErrSet_Constant1 ==
  MmAxis_in : Inport
  ErrSwitch : Inport  Port=2
  MmAxis_Num : Inport  Port=3
  Compare To Zero : simulink/Logic and Bit Operations/Compare To Zero  relop===  OutDataTypeStr=boolean
  Demux1 : Demux  Outputs=2
  Logical Operator : Logic  Operator=OR  AllPortsSameDT=off  OutDataTypeStr=boolean
  Memory : Memory
  Relational Operator9 : RelationalOperator  Operator===  OutDataTypeStr=boolean  RndMeth=Simplest
  Switch1 : Switch  Criteria=u2 > Threshold  Threshold=0.5
  Triggered Subsystem8 : Subsystem  TreatAsAtomicUnit=on
  MmAxis_out : Outport
  wires:
  Logical Operator/1 -> Triggered Subsystem8/Enable
  Compare To Zero/1 -> Logical Operator/1
  Relational Operator9/1 -> Logical Operator/2
  MmAxis_Num/1 -> Relational Operator9/1
  Demux1/1 -> Relational Operator9/2, Compare To Zero/1
  Triggered Subsystem8/1(Out1) -> Switch1/2
  ErrSwitch/1 -> Demux1/1
  Memory/1 -> Switch1/1
  Demux1/2 -> Triggered Subsystem8/1(In1)
  MmAxis_in/1 -> Switch1/3
  Switch1/1 -> Memory/1, MmAxis_out/1

== system GS_model/Subsystem2/Subsystem/Sensor/Magnetometer/MmModel3/Mm_ErrSet/MmErrSet/MmErrSet_Constant/MmAxisXErrSet_Constant2 ==
  MmAxis_in : Inport
  ErrSwitch : Inport  Port=2
  MmAxis_Num : Inport  Port=3
  Compare To Zero : simulink/Logic and Bit Operations/Compare To Zero  relop===  OutDataTypeStr=boolean
  Demux1 : Demux  Outputs=2
  Logical Operator : Logic  Operator=OR  AllPortsSameDT=off  OutDataTypeStr=boolean
  Memory : Memory
  Relational Operator9 : RelationalOperator  Operator===  OutDataTypeStr=boolean  RndMeth=Simplest
  Switch1 : Switch  Criteria=u2 > Threshold  Threshold=0.5
  Triggered Subsystem8 : Subsystem  TreatAsAtomicUnit=on
  MmAxis_out : Outport
  wires:
  Switch1/1 -> MmAxis_out/1, Memory/1
  MmAxis_in/1 -> Switch1/3
  Demux1/2 -> Triggered Subsystem8/1(In1)
  Memory/1 -> Switch1/1
  ErrSwitch/1 -> Demux1/1
  Triggered Subsystem8/1(Out1) -> Switch1/2
  Demux1/1 -> Compare To Zero/1, Relational Operator9/2
  MmAxis_Num/1 -> Relational Operator9/1
  Relational Operator9/1 -> Logical Operator/2
  Compare To Zero/1 -> Logical Operator/1
  Logical Operator/1 -> Triggered Subsystem8/Enable

== system GS_model/Subsystem2/Subsystem/Sensor/Magnetometer/MmModel3/Mm_ErrSet/MmErrSet/MmErrSet_Jump/MmAxisXErrSet_Jump ==
  MmAxis_in : Inport
  ErrSet : Inport  Port=2
  MmAxis_Num : Inport  Port=3
  MmAxis_JumpSet : Inport  Port=4
  Add : Sum  Inputs=|++
  Compare To Zero : simulink/Logic and Bit Operations/Compare To Zero  relop===  OutDataTypeStr=boolean
  Demux1 : Demux
  Logical Operator : Logic  Operator=OR  AllPortsSameDT=off  OutDataTypeStr=boolean
  Product : Product
  Relational Operator9 : RelationalOperator  Operator===  OutDataTypeStr=boolean  RndMeth=Simplest
  Switch3 : Switch  Criteria=u2 > Threshold  Threshold=0.5
  Terminator : Terminator
  Triggered Subsystem8 : Subsystem  TreatAsAtomicUnit=on
  MmAxis_out : Outport
  wires:
  MmAxis_JumpSet/1 -> Product/1
  Switch3/1 -> MmAxis_out/1
  MmAxis_Num/1 -> Relational Operator9/2
  Demux1/3 -> Terminator/1  "Period"
  Add/1 -> Switch3/1
  ErrSet/1 -> Demux1/1
  MmAxis_in/1 -> Add/2, Switch3/3
  Demux1/2 -> Triggered Subsystem8/1(In1)  "Switch"
  Product/1 -> Add/1
  Triggered Subsystem8/1(Out1) -> Switch3/2
  Demux1/4 -> Product/2  "Coff"
  Demux1/1 -> Compare To Zero/1, Relational Operator9/1  "Axis"
  Relational Operator9/1 -> Logical Operator/2
  Compare To Zero/1 -> Logical Operator/1
  Logical Operator/1 -> Triggered Subsystem8/Enable

== system GS_model/Subsystem2/Subsystem/Sensor/Magnetometer/MmModel3/Mm_ErrSet/MmErrSet/MmErrSet_Jump/MmAxisXErrSet_Jump1 ==
  MmAxis_in : Inport
  ErrSet : Inport  Port=2
  MmAxis_Num : Inport  Port=3
  MmAxis_JumpSet : Inport  Port=4
  Add : Sum  Inputs=|++
  Compare To Zero : simulink/Logic and Bit Operations/Compare To Zero  relop===  OutDataTypeStr=boolean
  Demux1 : Demux
  Logical Operator : Logic  Operator=OR  AllPortsSameDT=off  OutDataTypeStr=boolean
  Product : Product
  Relational Operator9 : RelationalOperator  Operator===  OutDataTypeStr=boolean  RndMeth=Simplest
  Switch3 : Switch  Criteria=u2 > Threshold  Threshold=0.5
  Terminator : Terminator
  Triggered Subsystem8 : Subsystem  TreatAsAtomicUnit=on
  MmAxis_out : Outport
  wires:
  Logical Operator/1 -> Triggered Subsystem8/Enable
  Compare To Zero/1 -> Logical Operator/1
  Relational Operator9/1 -> Logical Operator/2
  Demux1/1 -> Relational Operator9/1, Compare To Zero/1  "Axis"
  Demux1/4 -> Product/2  "Coff"
  Triggered Subsystem8/1(Out1) -> Switch3/2
  Product/1 -> Add/1
  Demux1/2 -> Triggered Subsystem8/1(In1)  "Switch"
  MmAxis_in/1 -> Switch3/3, Add/2
  ErrSet/1 -> Demux1/1
  Add/1 -> Switch3/1
  Demux1/3 -> Terminator/1  "Period"
  MmAxis_Num/1 -> Relational Operator9/2
  Switch3/1 -> MmAxis_out/1
  MmAxis_JumpSet/1 -> Product/1

== system GS_model/Subsystem2/Subsystem/Sensor/Magnetometer/MmModel3/Mm_ErrSet/MmErrSet/MmErrSet_Jump/MmAxisXErrSet_Jump2 ==
  MmAxis_in : Inport
  ErrSet : Inport  Port=2
  MmAxis_Num : Inport  Port=3
  MmAxis_JumpSet : Inport  Port=4
  Add : Sum  Inputs=|++
  Compare To Zero : simulink/Logic and Bit Operations/Compare To Zero  relop===  OutDataTypeStr=boolean
  Demux1 : Demux
  Logical Operator : Logic  Operator=OR  AllPortsSameDT=off  OutDataTypeStr=boolean
  Product : Product
  Relational Operator9 : RelationalOperator  Operator===  OutDataTypeStr=boolean  RndMeth=Simplest
  Switch3 : Switch  Criteria=u2 > Threshold  Threshold=0.5
  Terminator : Terminator
  Triggered Subsystem8 : Subsystem  TreatAsAtomicUnit=on
  MmAxis_out : Outport
  wires:
  MmAxis_JumpSet/1 -> Product/1
  Switch3/1 -> MmAxis_out/1
  MmAxis_Num/1 -> Relational Operator9/2
  Demux1/3 -> Terminator/1  "Period"
  Add/1 -> Switch3/1
  ErrSet/1 -> Demux1/1
  MmAxis_in/1 -> Add/2, Switch3/3
  Demux1/2 -> Triggered Subsystem8/1(In1)  "Switch"
  Product/1 -> Add/1
  Triggered Subsystem8/1(Out1) -> Switch3/2
  Demux1/4 -> Product/2  "Coff"
  Demux1/1 -> Compare To Zero/1, Relational Operator9/1  "Axis"
  Relational Operator9/1 -> Logical Operator/2
  Compare To Zero/1 -> Logical Operator/1
  Logical Operator/1 -> Triggered Subsystem8/Enable

== system GS_model/Subsystem2/Subsystem/Sensor/Magnetometer/MmModel3/Mm_ErrSet/MmErrSet/MmErrSet_Wave/MmAxisXErrSet_Wave ==
  MmAxis_in : Inport
  ErrSet : Inport  Port=2
  MmAxis_Num : Inport  Port=3
  MmAxis_WaveSet : Inport  Port=4
  Add : Sum  Inputs=|++
  Compare To Zero : simulink/Logic and Bit Operations/Compare To Zero  relop===  OutDataTypeStr=boolean
  Demux1 : Demux  Outputs=3
  Logical Operator : Logic  Operator=OR  AllPortsSameDT=off  OutDataTypeStr=boolean
  Product : Product
  Relational Operator9 : RelationalOperator  Operator===  OutDataTypeStr=boolean  RndMeth=Simplest
  Switch3 : Switch  Criteria=u2 > Threshold  Threshold=0.5
  Triggered Subsystem8 : Subsystem  TreatAsAtomicUnit=on
  MmAxis_out : Outport
  wires:
  Triggered Subsystem8/1(Out1) -> Switch3/2
  Switch3/1 -> MmAxis_out/1
  MmAxis_Num/1 -> Relational Operator9/2
  Demux1/3 -> Product/2  "Coff"
  Demux1/1 -> Compare To Zero/1, Relational Operator9/1  "Axis"
  Demux1/2 -> Triggered Subsystem8/1(In1)  "Switch"
  MmAxis_in/1 -> Switch3/3, Add/2
  Add/1 -> Switch3/1
  ErrSet/1 -> Demux1/1
  Product/1 -> Add/1
  MmAxis_WaveSet/1 -> Product/1
  Relational Operator9/1 -> Logical Operator/2
  Logical Operator/1 -> Triggered Subsystem8/Enable
  Compare To Zero/1 -> Logical Operator/1

== system GS_model/Subsystem2/Subsystem/Sensor/Magnetometer/MmModel3/Mm_ErrSet/MmErrSet/MmErrSet_Wave/MmAxisXErrSet_Wave1 ==
  MmAxis_in : Inport
  ErrSet : Inport  Port=2
  MmAxis_Num : Inport  Port=3
  MmAxis_WaveSet : Inport  Port=4
  Add : Sum  Inputs=|++
  Compare To Zero : simulink/Logic and Bit Operations/Compare To Zero  relop===  OutDataTypeStr=boolean
  Demux1 : Demux  Outputs=3
  Logical Operator : Logic  Operator=OR  AllPortsSameDT=off  OutDataTypeStr=boolean
  Product : Product
  Relational Operator9 : RelationalOperator  Operator===  OutDataTypeStr=boolean  RndMeth=Simplest
  Switch3 : Switch  Criteria=u2 > Threshold  Threshold=0.5
  Triggered Subsystem8 : Subsystem  TreatAsAtomicUnit=on
  MmAxis_out : Outport
  wires:
  Compare To Zero/1 -> Logical Operator/1
  Logical Operator/1 -> Triggered Subsystem8/Enable
  Relational Operator9/1 -> Logical Operator/2
  MmAxis_WaveSet/1 -> Product/1
  Product/1 -> Add/1
  ErrSet/1 -> Demux1/1
  Add/1 -> Switch3/1
  MmAxis_in/1 -> Add/2, Switch3/3
  Demux1/2 -> Triggered Subsystem8/1(In1)  "Switch"
  Demux1/1 -> Relational Operator9/1, Compare To Zero/1  "Axis"
  Demux1/3 -> Product/2  "Coff"
  MmAxis_Num/1 -> Relational Operator9/2
  Switch3/1 -> MmAxis_out/1
  Triggered Subsystem8/1(Out1) -> Switch3/2

== system GS_model/Subsystem2/Subsystem/Sensor/Magnetometer/MmModel3/Mm_ErrSet/MmErrSet/MmErrSet_Wave/MmAxisXErrSet_Wave2 ==
  MmAxis_in : Inport
  ErrSet : Inport  Port=2
  MmAxis_Num : Inport  Port=3
  MmAxis_WaveSet : Inport  Port=4
  Add : Sum  Inputs=|++
  Compare To Zero : simulink/Logic and Bit Operations/Compare To Zero  relop===  OutDataTypeStr=boolean
  Demux1 : Demux  Outputs=3
  Logical Operator : Logic  Operator=OR  AllPortsSameDT=off  OutDataTypeStr=boolean
  Product : Product
  Relational Operator9 : RelationalOperator  Operator===  OutDataTypeStr=boolean  RndMeth=Simplest
  Switch3 : Switch  Criteria=u2 > Threshold  Threshold=0.5
  Triggered Subsystem8 : Subsystem  TreatAsAtomicUnit=on
  MmAxis_out : Outport
  wires:
  Triggered Subsystem8/1(Out1) -> Switch3/2
  Switch3/1 -> MmAxis_out/1
  MmAxis_Num/1 -> Relational Operator9/2
  Demux1/3 -> Product/2  "Coff"
  Demux1/1 -> Compare To Zero/1, Relational Operator9/1  "Axis"
  Demux1/2 -> Triggered Subsystem8/1(In1)  "Switch"
  MmAxis_in/1 -> Switch3/3, Add/2
  Add/1 -> Switch3/1
  ErrSet/1 -> Demux1/1
  Product/1 -> Add/1
  MmAxis_WaveSet/1 -> Product/1
  Relational Operator9/1 -> Logical Operator/2
  Logical Operator/1 -> Triggered Subsystem8/Enable
  Compare To Zero/1 -> Logical Operator/1

== system GS_model/Subsystem2/Subsystem/Sensor/Magnetometer/MmModel3/Mm_ErrSet/MmErrSet/MmErrSet_WildValue/MmAxisXErrSet_WildValue ==
  MmAxis_in : Inport
  ErrSwitch : Inport  Port=2
  MmAxis_Num : Inport  Port=3
  MmAxis_WildValue : Inport  Port=4
  Compare To Zero : simulink/Logic and Bit Operations/Compare To Zero  relop===  OutDataTypeStr=boolean
  Demux1 : Demux  Outputs=2
  Logical Operator : Logic  Operator=OR  AllPortsSameDT=off  OutDataTypeStr=boolean
  Relational Operator9 : RelationalOperator  Operator===  OutDataTypeStr=boolean  RndMeth=Simplest
  Switch1 : Switch  Criteria=u2 > Threshold  Threshold=0.5
  Triggered Subsystem8 : Subsystem  TreatAsAtomicUnit=on
  MmAxis_out : Outport
  wires:
  ErrSwitch/1 -> Demux1/1
  MmAxis_WildValue/1 -> Switch1/1
  MmAxis_Num/1 -> Relational Operator9/2
  Triggered Subsystem8/1(Out1) -> Switch1/2
  Demux1/2 -> Triggered Subsystem8/1(In1)
  Demux1/1 -> Compare To Zero/1, Relational Operator9/1
  MmAxis_in/1 -> Switch1/3
  Switch1/1 -> MmAxis_out/1
  Relational Operator9/1 -> Logical Operator/2
  Compare To Zero/1 -> Logical Operator/1
  Logical Operator/1 -> Triggered Subsystem8/Enable
